simulink model "DTM_sim"  (R2024b)
settings: Solver=ode3  StartTime=0.0  StopTime=time_simulated  FixedStep=time_step_size  RelTol=1e-3
values from neighbouring files (symbols this model uses):
  a = 0.276626506024    [Fufy.mat]    (also in STMDrift.m = 1.347; Trajectory_LQR_double_track_Workspace_Phase_Plane_16_06.m = l-b; initParam.m = l-b)
  Ackerman_front = 0    [Fufy.mat]
  Ackerman_rear = 0    [Fufy.mat]
  b = 0.283373493976    [Fufy.mat]    (also in STMDrift.m = 1.393; Trajectory_LQR_double_track_Workspace_Phase_Plane_16_06.m = l/2; initParam.m = l/2)
  constant_force = 9    [runSIM.m]
  constant_steer = deg2rad(15)    [runSIM.m]
  d = 0    [Fufy.mat]
  d_front = 0    [Fufy.mat]
  d_rear = 0    [Fufy.mat]
  g = 9.81    [Fufy.mat]    (also in STMDrift.m)
  gamma = pi/2    (= 1.57079632679)    [Trajectory_LQR_double_track_Workspace_Phase_Plane_16_06.m]    (also in initParam.m; runSIM.m = 0)
  h = 0.128945128333    [Fufy.mat]    (also in STMDrift.m = [v;       beta;       d_delta;       d_Fx]; Trajectory_LQR_double_track_Workspace_Phase_Plane_16_06.m = (Fz_rear*l/(Fz_Tot)-(l-b))*cot(asin(H/l))+(R_r+R_f)/2; initParam.m = (Fz_Rear*l/(Fz_Tot)-(l-b))*cot(asin(H/l))+(R_r+R_f)/2)
  I_wheel = 0.002933125    [Fufy.mat]
  J_CoG = 1.30125108434    [Fufy.mat]    (also in Trajectory_LQR_double_track_Workspace_Phase_Plane_16_06.m = 9.4*a^2+9.4*b^2; initParam.m = 9.4*a^2+9.4*b^2)
  k_roll_front = 1    [Fufy.mat]
  k_roll_rear = 1    [Fufy.mat]
  l = 0.56    [Fufy.mat]
  m = 16.6    [Fufy.mat]    (also in STMDrift.m = 2137.3; Trajectory_LQR_double_track_Workspace_Phase_Plane_16_06.m = 18.8; initParam.m = 18.8)
  R_f = 0.095    [Fufy.mat]
  R_fl = R_f    [Trajectory_LQR_double_track_Workspace_Phase_Plane_16_06.m]    (also in initParam.m)
  R_fr = R_f    [Trajectory_LQR_double_track_Workspace_Phase_Plane_16_06.m]    (also in initParam.m)
  R_r = 0.095    [Fufy.mat]
  R_rl = R_r    [Trajectory_LQR_double_track_Workspace_Phase_Plane_16_06.m]    (also in initParam.m)
  R_rr = R_r    [Trajectory_LQR_double_track_Workspace_Phase_Plane_16_06.m]    (also in initParam.m)
  steering_ratio_f = 0.6    [Fufy.mat]
  steering_ratio_r = 0    [Fufy.mat]
  t_front = t    [Trajectory_LQR_double_track_Workspace_Phase_Plane_16_06.m]    (also in initParam.m)
  t_rear = t    [Trajectory_LQR_double_track_Workspace_Phase_Plane_16_06.m]    (also in initParam.m)
  Toe_fl = -0*pi/180    (= 0)    [Trajectory_LQR_double_track_Workspace_Phase_Plane_16_06.m]    (also in initParam.m)
  Toe_fr = -Toe_fl    (= 0)    [Trajectory_LQR_double_track_Workspace_Phase_Plane_16_06.m]    (also in initParam.m)
  Toe_rl = 0*pi/180    (= 0)    [Trajectory_LQR_double_track_Workspace_Phase_Plane_16_06.m]    (also in initParam.m)
  Toe_rr = -Toe_rl    (= 0)    [Trajectory_LQR_double_track_Workspace_Phase_Plane_16_06.m]    (also in initParam.m)
  u0 = 0    [Trajectory_LQR_double_track_Workspace_Phase_Plane_16_06.m]    (also in runSIM.m = 1)
  v0 = 0    [Trajectory_LQR_double_track_Workspace_Phase_Plane_16_06.m]    (also in runSIM.m = 8)
  yaw_rate0 = 0    [Trajectory_LQR_double_track_Workspace_Phase_Plane_16_06.m]    (also in runSIM.m = deg2rad(15))
undefined symbols (not defined in the file or in its folder): angular_speed_fl0, angular_speed_fr0, angular_speed_rl0, angular_speed_rr0, Fz_fl, Fz_fr, Fz_rl, Fz_rr
libraries: simulink_extras x1
settings Model: Creator=pc  LastModifiedBy=mg

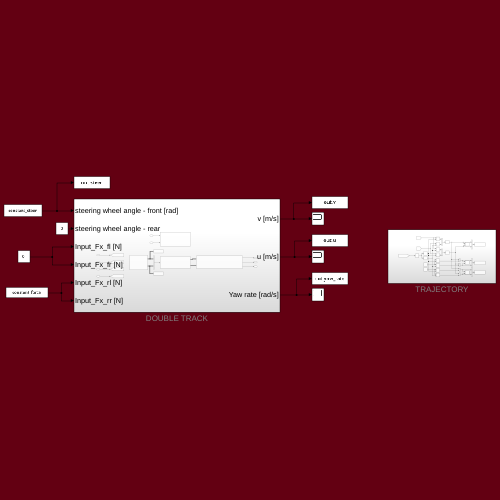
[thumbnail: Simulink's stored preview of the top-level diagram]
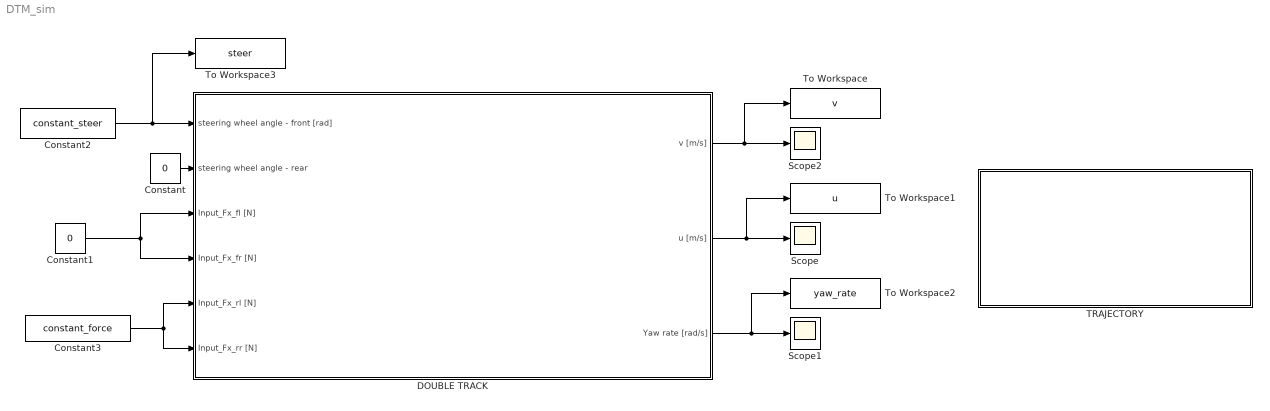
== system DTM_sim ==
  Constant : Constant  Value=0
  Constant1 : Constant  Value=0
  Constant2 : Constant  Value=constant_steer
  Constant3 : Constant  Value=constant_force
  DOUBLE TRACK : Subsystem
  Scope : Scope
  Scope1 : Scope
  Scope2 : Scope
  TRAJECTORY : Subsystem
  To Workspace : ToWorkspace  VariableName=v  SampleTime=-1
  To Workspace1 : ToWorkspace  VariableName=u  SampleTime=-1
  To Workspace2 : ToWorkspace  VariableName=yaw_rate  SampleTime=-1
  To Workspace3 : ToWorkspace  VariableName=steer  SampleTime=-1
  wires:
  Constant/1 -> DOUBLE TRACK/2(steering wheel angle - rear)
  Constant1/1 -> DOUBLE TRACK/4(Input_Fx_fr [N]), DOUBLE TRACK/3(Input_Fx_fl [N])
  DOUBLE TRACK/2(u [m/s]) -> To Workspace1/1, Scope/1
  DOUBLE TRACK/3(Yaw rate [rad/s]) -> To Workspace2/1, Scope1/1
  DOUBLE TRACK/1(v [m/s]) -> To Workspace/1, Scope2/1
  Constant2/1 -> To Workspace3/1, DOUBLE TRACK/1(steering wheel angle - front [rad])
  Constant3/1 -> DOUBLE TRACK/6(Input_Fx_rr [N]), DOUBLE TRACK/5(Input_Fx_rl [N])

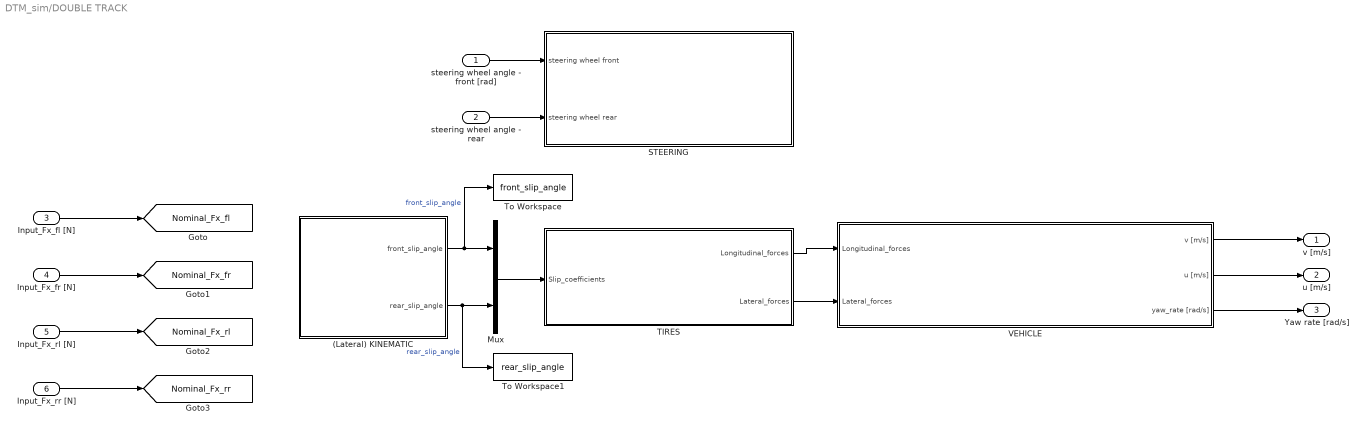
== system DTM_sim/DOUBLE TRACK ==
  steering wheel angle - front [rad] : Inport
  steering wheel angle - rear : Inport  Port=2
  Input_Fx_fl [N] : Inport  Port=3
  Input_Fx_fr [N] : Inport  Port=4
  Input_Fx_rl [N] : Inport  Port=5
  Input_Fx_rr [N] : Inport  Port=6
  (Lateral) KINEMATIC : Subsystem
  Mux : Mux  Inputs=2
  STEERING : Subsystem
  TIRES : Subsystem
  To Workspace : ToWorkspace  VariableName=front_slip_angle  SampleTime=-1
  To Workspace1 : ToWorkspace  VariableName=rear_slip_angle  SampleTime=-1
  VEHICLE : Subsystem
  v [m/s] : Outport
  u [m/s] : Outport  Port=2
  Yaw rate [rad/s] : Outport  Port=3
  tag scope: Nominal_Fx_fl=global, Nominal_Fx_fr=global, Nominal_Fx_rl=global, Nominal_Fx_rr=global
  wires:
  steering wheel angle - front [rad]/1 -> STEERING/1(steering wheel front)
  steering wheel angle - rear/1 -> STEERING/2(steering wheel rear)
  Input_Fx_fl [N]/1 -> [Nominal_Fx_fl]
  Input_Fx_fr [N]/1 -> [Nominal_Fx_fr]
  Input_Fx_rl [N]/1 -> [Nominal_Fx_rl]
  Input_Fx_rr [N]/1 -> [Nominal_Fx_rr]
  (Lateral) KINEMATIC/2(rear_slip_angle) -> To Workspace1/1, Mux/2  "rear_slip_angle"
  (Lateral) KINEMATIC/1(front_slip_angle) -> To Workspace/1, Mux/1  "front_slip_angle"
  Mux/1 -> TIRES/1(Slip_coefficients)
  TIRES/1(Longitudinal_forces) -> VEHICLE/1(Longitudinal_forces)
  TIRES/2(Lateral_forces) -> VEHICLE/2(Lateral_forces)
  VEHICLE/3(yaw_rate [rad/s]) -> Yaw rate [rad/s]/1
  VEHICLE/2(u [m/s]) -> u [m/s]/1
  VEHICLE/1(v [m/s]) -> v [m/s]/1

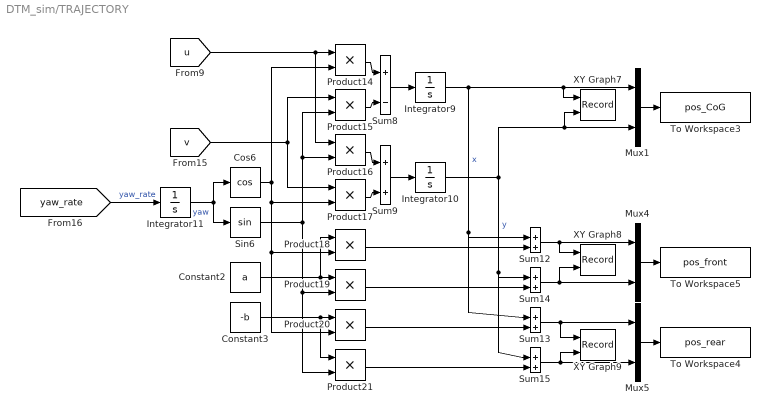
== system DTM_sim/TRAJECTORY ==
  Constant2 : Constant  Value=a
  Constant3 : Constant  Value=-b
  Cos6 : Trigonometry  Operator=cos
  Integrator10 : Integrator  InitialCondition=v0
  Integrator11 : Integrator  InitialCondition=gamma
  Integrator9 : Integrator  InitialCondition=u0
  Mux1 : Mux  Inputs=2
  Mux4 : Mux  Inputs=2
  Mux5 : Mux  Inputs=2
  Product{14..21} (8 alike) : Product
  Sin6 : Trigonometry
  Sum{9,12..15} (5 alike) : Sum  Inputs=+||+
  Sum8 : Sum  Inputs=+||-
  To Workspace3 : ToWorkspace  VariableName=pos_CoG  SampleTime=-1
  To Workspace4 : ToWorkspace  VariableName=pos_rear  SampleTime=-1
  To Workspace5 : ToWorkspace  VariableName=pos_front  SampleTime=-1
  XY Graph7 : Record  FileSettingsInternal="{\"entries\":[{\"content\":{\"excelSettings\":{\"content\":{},\"type\":\"Streamout.ExcelSettings\"}},\"type\":\"Streamout.FileSettingStorage\",\"uuid\":\"\"}],\"packageUris\":[\"http:\\/\\/schema.mathworks.com\\/mf0\\/streamout_blocks\\/R2020a\"],\"version\":\"1.0\"}"  Layout=[1 1]  SignalsInternal="{\"entries\":[{\"content\":{\"signals\":[{\"content\":{\"blockPath\":[],\"dimensions\":[1],\"domain\":\"\",\"lineColor\":\"#64d413\",\"lineWidth\":2,\"port\":1,\"signalID\":1,\"signalName\":\"MATLAB Function1\"},\"type\":\"RecordBlkView.Signal\",\"uuid\":\"\"},{\"content\":{\"blockPath\":[],\"dimensions\":[1],\"domain\":\"\",\"lineColor\":\"#ff13a6\",\"lineWidth\":2,\"port\":2,\"signalID\":2,\"signalName\":\"MATLAB Function\"},\"type\":\"RecordBlkView.Signal\",\"uuid\":\"\"}]},\"type\":\"RecordBlkView.InputSignals\",\"uuid\":\"\"}],\"packageUris\":[\"http:\\/\\/schema.mathworks.com\\/mf0\\/streamout_blocks\\/R2020a\"],\"version\":\"1.0\"}"  VisualizationBindings="{\"xyplotplugin\":{\"info\":[{\"series\":[],\"subplotID\":1}]}}"  CompatibilityTag=XY
  XY Graph8 : Record  FileSettingsInternal="{\"entries\":[{\"content\":{\"excelSettings\":{\"content\":{},\"type\":\"Streamout.ExcelSettings\"}},\"type\":\"Streamout.FileSettingStorage\",\"uuid\":\"\"}],\"packageUris\":[\"http:\\/\\/schema.mathworks.com\\/mf0\\/streamout_blocks\\/R2020a\"],\"version\":\"1.0\"}"  Layout=[1 1]  SignalsInternal="{\"entries\":[{\"content\":{\"signals\":[{\"content\":{\"blockPath\":[],\"dimensions\":[1],\"domain\":\"\",\"lineColor\":\"#64d413\",\"lineWidth\":2,\"port\":1,\"signalID\":1,\"signalName\":\"MATLAB Function1\"},\"type\":\"RecordBlkView.Signal\",\"uuid\":\"\"},{\"content\":{\"blockPath\":[],\"dimensions\":[1],\"domain\":\"\",\"lineColor\":\"#ff13a6\",\"lineWidth\":2,\"port\":2,\"signalID\":2,\"signalName\":\"MATLAB Function\"},\"type\":\"RecordBlkView.Signal\",\"uuid\":\"\"}]},\"type\":\"RecordBlkView.InputSignals\",\"uuid\":\"\"}],\"packageUris\":[\"http:\\/\\/schema.mathworks.com\\/mf0\\/streamout_blocks\\/R2020a\"],\"version\":\"1.0\"}"  VisualizationBindings="{\"xyplotplugin\":{\"info\":[{\"series\":[],\"subplotID\":1}]}}"  CompatibilityTag=XY
  XY Graph9 : Record  FileSettingsInternal="{\"entries\":[{\"content\":{\"excelSettings\":{\"content\":{},\"type\":\"Streamout.ExcelSettings\"}},\"type\":\"Streamout.FileSettingStorage\",\"uuid\":\"\"}],\"packageUris\":[\"http:\\/\\/schema.mathworks.com\\/mf0\\/streamout_blocks\\/R2020a\"],\"version\":\"1.0\"}"  Layout=[1 1]  SignalsInternal="{\"entries\":[{\"content\":{\"signals\":[{\"content\":{\"blockPath\":[],\"dimensions\":[1],\"domain\":\"\",\"lineColor\":\"#64d413\",\"lineWidth\":2,\"port\":1,\"signalID\":1,\"signalName\":\"MATLAB Function1\"},\"type\":\"RecordBlkView.Signal\",\"uuid\":\"\"},{\"content\":{\"blockPath\":[],\"dimensions\":[1],\"domain\":\"\",\"lineColor\":\"#ff13a6\",\"lineWidth\":2,\"port\":2,\"signalID\":2,\"signalName\":\"MATLAB Function\"},\"type\":\"RecordBlkView.Signal\",\"uuid\":\"\"}]},\"type\":\"RecordBlkView.InputSignals\",\"uuid\":\"\"}],\"packageUris\":[\"http:\\/\\/schema.mathworks.com\\/mf0\\/streamout_blocks\\/R2020a\"],\"version\":\"1.0\"}"  VisualizationBindings="{\"xyplotplugin\":{\"info\":[{\"series\":[],\"subplotID\":1}]}}"  CompatibilityTag=XY
  wires:
  Mux4/1 -> To Workspace5/1
  Mux5/1 -> To Workspace4/1
  Sum13/1 -> Mux5/1, XY Graph9/1
  Sum15/1 -> Mux5/2, XY Graph9/2
  Sum14/1 -> XY Graph8/2, Mux4/2
  Sum12/1 -> Mux4/1, XY Graph8/1
  Constant3/1 -> Product20/1, Product21/1
  Constant2/1 -> Product18/1, Product19/1
  Product20/1 -> Sum13/2
  Product21/1 -> Sum15/2
  Product19/1 -> Sum14/2
  Product18/1 -> Sum12/2
  Mux1/1 -> To Workspace3/1
  Sum9/1 -> Integrator10/1
  Sum8/1 -> Integrator9/1
  [v] -> Product17/1, Product15/1
  Product16/1 -> Sum9/1
  Product17/1 -> Sum9/2
  Product15/1 -> Sum8/2
  Sin6/1 -> Product19/2, Product21/2, Product15/2, Product16/2
  Product14/1 -> Sum8/1
  [u] -> Product14/1, Product16/1
  Cos6/1 -> Product14/2, Product17/2, Product18/2, Product20/2
  Integrator11/1 -> Cos6/1, Sin6/1  "yaw"
  Integrator10/1 -> Mux1/2, XY Graph7/2, Sum14/1, Sum15/1  "y"
  Integrator9/1 -> XY Graph7/1, Mux1/1, Sum12/1, Sum13/1  "x"
  [yaw_rate] -> Integrator11/1  "yaw_rate"

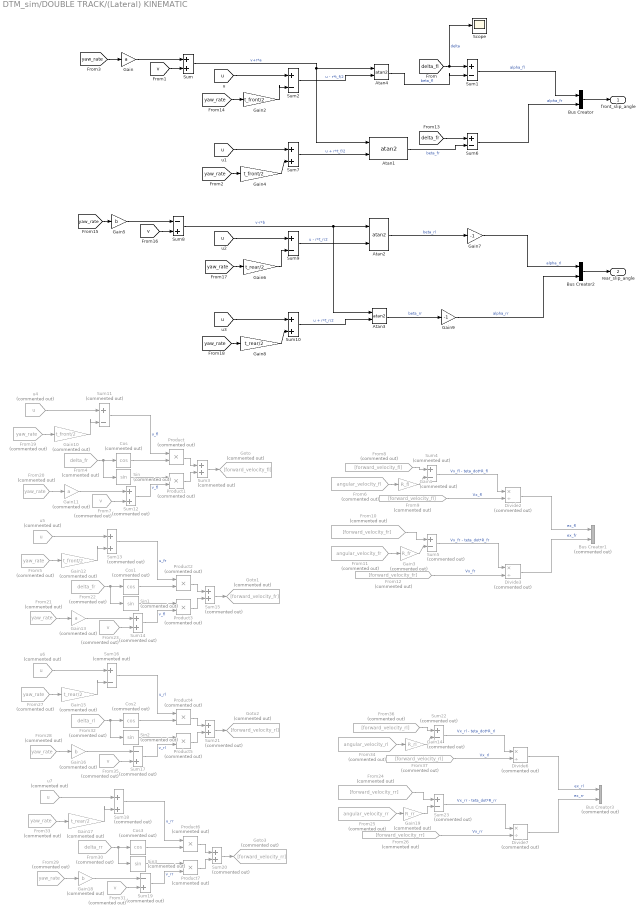
== system DTM_sim/DOUBLE TRACK/(Lateral) KINEMATIC ==
  Atan{1..4} (4 alike) : Trigonometry  Operator=atan2
  Bus Creator : BusCreator  Inputs=2
  Bus Creator1 : BusCreator  Commented=on  Inputs=2
  Bus Creator2 : BusCreator  Inputs=2
  Bus Creator3 : BusCreator  Commented=on  Inputs=2
  Cos{,1..3} (4 alike) : Trigonometry  Commented=on  Operator=cos
  Divide{2..3,6..7} (4 alike) : Product  Commented=on  Inputs=*/
  From10 : From  Commented=on  GotoTag=forward_velocity_fr
  From11 : From  Commented=on  GotoTag=angular_velocity_fr  TagVisibility=global
  From12 : From  Commented=on  GotoTag=forward_velocity_fr
  From{5,19..21,27..29,33} (8 alike) : From  Commented=on  GotoTag=yaw_rate  TagVisibility=global
  From22 : From  Commented=on  GotoTag=delta_fr  TagVisibility=global
  From{7,23,31,35} (4 alike) : From  Commented=on  GotoTag=v  TagVisibility=global
  From24 : From  Commented=on  GotoTag=forward_velocity_rr
  From25 : From  Commented=on  GotoTag=angular_velocity_rr  TagVisibility=global
  From26 : From  Commented=on  GotoTag=forward_velocity_rr
  From30 : From  Commented=on  GotoTag=delta_rr  TagVisibility=global
  From32 : From  Commented=on  GotoTag=delta_rl  TagVisibility=global
  From34 : From  Commented=on  GotoTag=angular_velocity_rl  TagVisibility=global
  From36 : From  Commented=on  GotoTag=forward_velocity_rl
  From37 : From  Commented=on  GotoTag=forward_velocity_rl
  From4 : From  Commented=on  GotoTag=delta_fr  TagVisibility=global
  From6 : From  Commented=on  GotoTag=angular_velocity_fl  TagVisibility=global
  From8 : From  Commented=on  GotoTag=forward_velocity_fl
  From9 : From  Commented=on  GotoTag=forward_velocity_fl
  Gain : Gain  Gain=a
  Gain1 : Gain  Commented=on  Gain=R_fl
  Gain10 : Gain  Commented=on  Gain=t_front/2
  Gain11 : Gain  Commented=on  Gain=a
  Gain12 : Gain  Commented=on  Gain=t_front/2
  Gain13 : Gain  Commented=on  Gain=a
  Gain14 : Gain  Commented=on  Gain=R_rl
  Gain15 : Gain  Commented=on  Gain=t_rear/2
  Gain16 : Gain  Commented=on  Gain=b
  Gain17 : Gain  Commented=on  Gain=t_rear/2
  Gain18 : Gain  Commented=on  Gain=b
  Gain19 : Gain  Commented=on  Gain=R_rr
  Gain2 : Gain  Gain=t_front/2
  Gain3 : Gain  Commented=on  Gain=R_fr
  Gain4 : Gain  Gain=t_front/2
  Gain5 : Gain  Gain=b
  Gain6 : Gain  Gain=t_rear/2
  Gain7 : Gain  Gain=-1
  Gain8 : Gain  Gain=t_rear/2
  Gain9 : Gain  Gain=-1
  Goto : Goto  Commented=on  GotoTag=forward_velocity_fl
  Goto1 : Goto  Commented=on  GotoTag=forward_velocity_fr
  Goto2 : Goto  Commented=on  GotoTag=forward_velocity_rl
  Goto3 : Goto  Commented=on  GotoTag=forward_velocity_rr
  Product{,1..7} (8 alike) : Product  Commented=on
  Scope : Scope
  Sin{,1..3} (4 alike) : Trigonometry  Commented=on
  Sum : Sum  Inputs=||+|||+||
  Sum1 : Sum  Inputs=||+||-||
  Sum10 : Sum  Inputs=||+|||+||
  Sum11 : Sum  Commented=on  Inputs=||+|||-||
  Sum{12..14,18} (4 alike) : Sum  Commented=on  Inputs=||+|||+||
  Sum{3,15,20..21} (4 alike) : Sum  Commented=on  Inputs=||+||+||
  Sum16 : Sum  Commented=on  Inputs=||+|||-||
  Sum17 : Sum  Commented=on  Inputs=||-|||+||
  Sum19 : Sum  Commented=on  Inputs=||-|||+||
  Sum2 : Sum  Inputs=||+|||-||
  Sum{4..5,22..23} (4 alike) : Sum  Commented=on  Inputs=||+||-||
  Sum6 : Sum  Inputs=||+||-||
  Sum7 : Sum  Inputs=||+|||+||
  Sum8 : Sum  Inputs=||-|||+||
  Sum9 : Sum  Inputs=||+|||-||
  u{4..7} (4 alike) : From  Commented=on  GotoTag=u  TagVisibility=global
  front_slip_angle : Outport
  rear_slip_angle : Outport  Port=2
  wires:
  Sum/1 -> Atan4/1, Atan1/1  "v+r*a"
  Atan4/1 -> Sum1/2  "beta_fl"
  [delta_fl] -> Scope/1, Sum1/1  "delta"
  [yaw_rate] -> Gain/1
  Atan1/1 -> Sum6/2  "beta_fr"
  Bus Creator/1 -> front_slip_angle/1
  Sum7/1 -> Atan1/2  "u + r*t_f/2"
  [v] -> Sum/2
  Gain/1 -> Sum/1
  From4/1 -> Sin/1, Cos/1
  Cos/1 -> Product/2
  Sin/1 -> Product1/1
  From6/1 -> Gain1/1
  Gain1/1 -> Sum4/2
  Sum4/1 -> Divide2/1  "Vx_fl - teta_dot*R_fl"
  Product1/1 -> Sum3/2
  Product/1 -> Sum3/1
  Sum3/1 -> Goto/1
  From8/1 -> Sum4/1
  From9/1 -> Divide2/2  "Vx_fl"
  Divide2/1 -> Bus Creator1/1  "ex_fl"
  Gain3/1 -> Sum5/2
  From11/1 -> Gain3/1
  From10/1 -> Sum5/1
  Sum5/1 -> Divide3/1  "Vx_fr - teta_dot*R_fr"
  From12/1 -> Divide3/2  "Vx_fr"
  Divide3/1 -> Bus Creator1/2  "ex_fr"
  Sum6/1 -> Bus Creator/2  "alpha_fr"
  [delta_fr] -> Sum6/1
  [u] -> Sum2/1
  Sum2/1 -> Atan4/2  "u - r*t_f/2"
  [yaw_rate] -> Gain2/1
  Gain2/1 -> Sum2/2
  [u] -> Sum7/1
  [yaw_rate] -> Gain4/1
  Gain4/1 -> Sum7/2
  [yaw_rate] -> Gain5/1
  Gain5/1 -> Sum8/1
  [v] -> Sum8/2
  Gain6/1 -> Sum9/2
  [u] -> Sum9/1
  [yaw_rate] -> Gain6/1
  Sum9/1 -> Atan2/2  "u - r*t_r/2"
  Atan2/1 -> Gain7/1  "beta_rl"
  Gain7/1 -> Bus Creator2/1  "alpha_rl"
  [u] -> Sum10/1
  Sum10/1 -> Atan3/2  "u + r*t_r/2"
  Sum8/1 -> Atan3/1, Atan2/1  "v-r*b"
  [yaw_rate] -> Gain8/1
  Gain8/1 -> Sum10/2
  Atan3/1 -> Gain9/1  "beta_rr"
  Gain9/1 -> Bus Creator2/2  "alpha_rr"
  Bus Creator2/1 -> rear_slip_angle/1
  u4/1 -> Sum11/1
  From19/1 -> Gain10/1
  Sum11/1 -> Product/1  "u_fl"
  Gain10/1 -> Sum11/2
  Gain11/1 -> Sum12/1
  From20/1 -> Gain11/1
  From7/1 -> Sum12/2
  Sum12/1 -> Product1/2  "v_fl"
  Sum14/1 -> Product3/2  "v_fl"
  Sum13/1 -> Product2/1  "u_fr"
  Gain12/1 -> Sum13/2
  u5/1 -> Sum13/1
  From23/1 -> Sum14/2
  Gain13/1 -> Sum14/1
  From21/1 -> Gain13/1
  Product3/1 -> Sum15/2
  Product2/1 -> Sum15/1
  From5/1 -> Gain12/1
  Sin1/1 -> Product3/1
  Sum15/1 -> Goto1/1
  Cos1/1 -> Product2/2
  From22/1 -> Sin1/1, Cos1/1
  Sum17/1 -> Product5/2  "v_rl"
  Sum16/1 -> Product4/1  "u_rl"
  Product7/1 -> Sum20/2
  From30/1 -> Sin3/1, Cos3/1
  From33/1 -> Gain17/1
  Sin3/1 -> Product7/1
  Cos3/1 -> Product6/2
  From29/1 -> Gain18/1
  Sum18/1 -> Product6/1  "u_rr"
  Sum20/1 -> Goto3/1
  u7/1 -> Sum18/1
  Gain17/1 -> Sum18/2
  Gain15/1 -> Sum16/2
  u6/1 -> Sum16/1
  From35/1 -> Sum17/2
  Gain18/1 -> Sum19/1
  Gain16/1 -> Sum17/1
  From28/1 -> Gain16/1
  From34/1 -> Gain14/1
  Sum22/1 -> Divide6/1  "Vx_rl - teta_dot*R_rl"
  Divide6/1 -> Bus Creator3/1  "ex_rl"
  From31/1 -> Sum19/2
  Cos2/1 -> Product4/2
  Sum23/1 -> Divide7/1  "Vx_rr - teta_dot*R_rr"
  From26/1 -> Divide7/2  "Vx_rr"
  Gain19/1 -> Sum23/2
  From37/1 -> Divide6/2  "Vx_rl"
  Divide7/1 -> Bus Creator3/2  "ex_rr"
  From24/1 -> Sum23/1
  Product5/1 -> Sum21/2
  From25/1 -> Gain19/1
  Product4/1 -> Sum21/1
  From27/1 -> Gain15/1
  Sin2/1 -> Product5/1
  Sum21/1 -> Goto2/1
  From36/1 -> Sum22/1
  Product6/1 -> Sum20/1
  From32/1 -> Sin2/1, Cos2/1
  Sum19/1 -> Product7/2  "v_rr"
  Gain14/1 -> Sum22/2
  Sum1/1 -> Bus Creator/1  "alpha_fl"

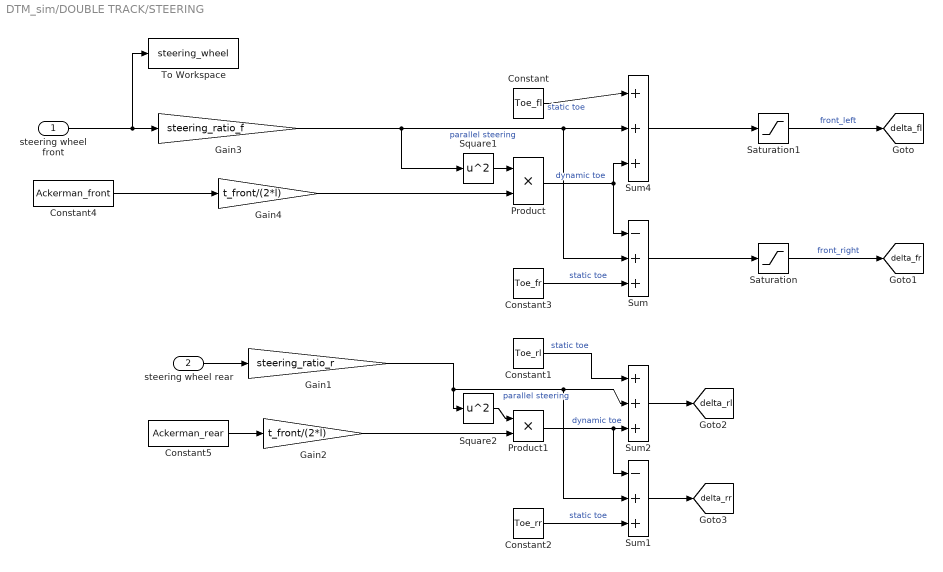
== system DTM_sim/DOUBLE TRACK/STEERING ==
  steering wheel front : Inport
  steering wheel rear : Inport  Port=2
  Constant : Constant  Value=Toe_fl
  Constant1 : Constant  Value=Toe_rl
  Constant2 : Constant  Value=Toe_rr
  Constant3 : Constant  Value=Toe_fr
  Constant4 : Constant  Value=Ackerman_front
  Constant5 : Constant  Value=Ackerman_rear
  Gain1 : Gain  Gain=steering_ratio_r
  Gain2 : Gain  Gain=t_front/(2*l)
  Gain3 : Gain  Gain=steering_ratio_f
  Gain4 : Gain  Gain=t_front/(2*l)
  Product : Product
  Product1 : Product
  Saturation : Saturate  UpperLimit=deg2rad(0.6*(84-47))  LowerLimit=deg2rad(0.6*(47-84))
  Saturation1 : Saturate  UpperLimit=deg2rad(0.6*(84-47))  LowerLimit=deg2rad(0.6*(47-84))
  Square1 : Math  Operator=square
  Square2 : Math  Operator=square
  Sum : Sum  Inputs=|-||||+||||+|
  Sum1 : Sum  Inputs=|-||||+||||+|
  Sum2 : Sum  Inputs=|+||||+||||+|
  Sum4 : Sum  Inputs=|+||||+||||+|
  To Workspace : ToWorkspace  VariableName=steering_wheel  SaveFormat=Structure With Time  SampleTime=-1
  tag scope: delta_fl=global, delta_fr=global, delta_rl=global, delta_rr=global
  wires:
  Constant4/1 -> Gain4/1
  Constant3/1 -> Sum/3  "static toe"
  Constant/1 -> Sum4/1  "static toe"
  steering wheel front/1 -> To Workspace/1, Gain3/1
  Product/1 -> Sum/1, Sum4/3  "dynamic toe"
  Gain3/1 -> Sum/2, Sum4/2, Square1/1  "parallel steering"
  Gain4/1 -> Product/2
  Square1/1 -> Product/1
  Constant1/1 -> Sum2/1  "static toe"
  Gain1/1 -> Square2/1, Sum1/2, Sum2/2  "parallel steering"
  steering wheel rear/1 -> Gain1/1
  Square2/1 -> Product1/1
  Sum1/1 -> [delta_rr]
  Product1/1 -> Sum1/1, Sum2/3  "dynamic toe"
  Gain2/1 -> Product1/2
  Sum2/1 -> [delta_rl]
  Constant5/1 -> Gain2/1
  Constant2/1 -> Sum1/3  "static toe"
  Sum4/1 -> Saturation1/1
  Saturation/1 -> [delta_fr]  "front_right"
  Saturation1/1 -> [delta_fl]  "front_left"
  Sum/1 -> Saturation/1

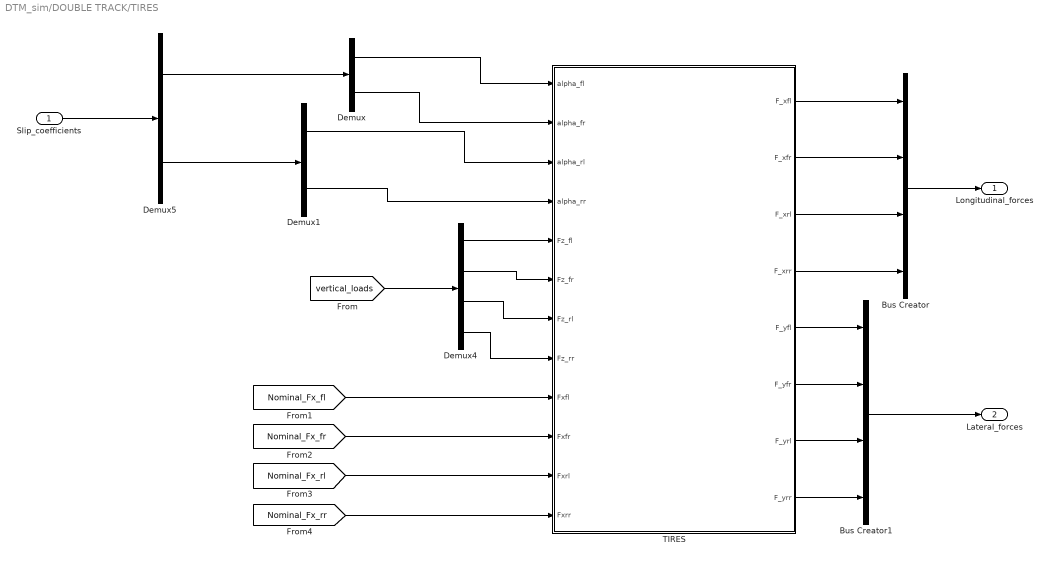
== system DTM_sim/DOUBLE TRACK/TIRES ==
  Slip_coefficients : Inport
  Bus Creator : BusCreator  Inputs=4
  Bus Creator1 : BusCreator  Inputs=4
  Demux : Demux  Outputs=2
  Demux1 : Demux  Outputs=2
  Demux4 : Demux
  Demux5 : Demux  Outputs=2
  TIRES : MATLAB Function  TreatAsAtomicUnit=on
  Longitudinal_forces : Outport
  Lateral_forces : Outport  Port=2
  wires:
  Bus Creator1/1 -> Lateral_forces/1
  Bus Creator/1 -> Longitudinal_forces/1
  Slip_coefficients/1 -> Demux5/1
  [vertical_loads] -> Demux4/1
  TIRES/1(F_xfl) -> Bus Creator/1
  TIRES/2(F_xfr) -> Bus Creator/2
  TIRES/3(F_xrl) -> Bus Creator/3
  TIRES/4(F_xrr) -> Bus Creator/4
  TIRES/5(F_yfl) -> Bus Creator1/1
  TIRES/6(F_yfr) -> Bus Creator1/2
  TIRES/7(F_yrl) -> Bus Creator1/3
  TIRES/8(F_yrr) -> Bus Creator1/4
  Demux/1 -> TIRES/1(alpha_fl)
  Demux/2 -> TIRES/2(alpha_fr)
  Demux1/1 -> TIRES/3(alpha_rl)
  Demux1/2 -> TIRES/4(alpha_rr)
  Demux4/1 -> TIRES/5(Fz_fl)
  Demux4/2 -> TIRES/6(Fz_fr)
  Demux4/3 -> TIRES/7(Fz_rl)
  Demux4/4 -> TIRES/8(Fz_rr)
  Demux5/2 -> Demux1/1
  Demux5/1 -> Demux/1
  [Nominal_Fx_fl] -> TIRES/9(Fxfl)
  [Nominal_Fx_fr] -> TIRES/10(Fxfr)
  [Nominal_Fx_rl] -> TIRES/11(Fxrl)
  [Nominal_Fx_rr] -> TIRES/12(Fxrr)

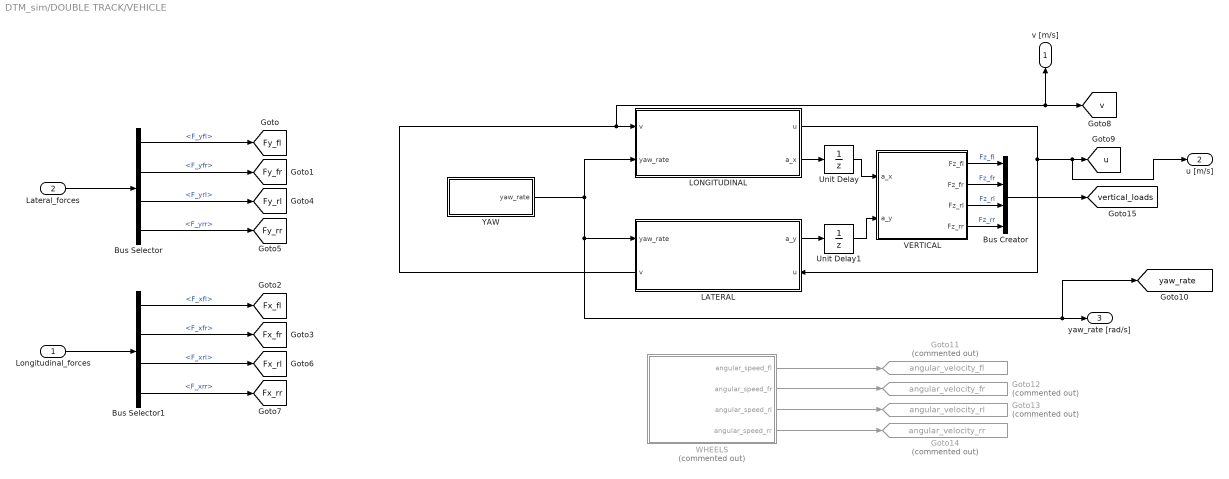
== system DTM_sim/DOUBLE TRACK/VEHICLE ==
  Longitudinal_forces : Inport
  Lateral_forces : Inport  Port=2
  Bus Creator : BusCreator  Inputs=Fz_fl,Fz_fr,Fz_rl,Fz_rr
  Bus Selector : BusSelector  OutputSignals=F_yfl,F_yfr,F_yrl,F_yrr
  Bus Selector1 : BusSelector  OutputSignals=F_xfl,F_xfr,F_xrl,F_xrr
  Goto11 : Goto  Commented=on  GotoTag=angular_velocity_fl  TagVisibility=global
  Goto12 : Goto  Commented=on  GotoTag=angular_velocity_fr  TagVisibility=global
  Goto13 : Goto  Commented=on  GotoTag=angular_velocity_rl  TagVisibility=global
  Goto14 : Goto  Commented=on  GotoTag=angular_velocity_rr  TagVisibility=global
  LATERAL : Subsystem
      settings: PortSchema="{\"entries\":[{\"content\":{\"sides\":[{\"content\":{\"connectorIds\":[\"In1\",\"Out2\"]},\"type\":\"ConnectorPlacement.EquallySpacedRectSide\",\"uuid\":\"6abf6559-6621-467b-b855-11099c66163f\"},{\"content\":{\"connectorIds\":[\"Out1\",\"In2\"],\"side\":\"RIGHT\"},\"type\":\"ConnectorPlacement.EquallySpacedRectSide\",\"uuid\":\"e2281ccf-38f1-4c2e-94ea-91f999c21e12\"},{\"content\":{\"side\":\"TOP\"},\"type\":\"ConnectorPlacement.EquallySpacedRectSide\",\"uuid\":\"84832623-c0ad-4def-a112-064fe8d35bcd\"}]},\"type\":\"ConnectorPlacement.EquallySpacedConnector\",\"uuid\":\"accfadac-0c65-44f3-8a84-674bad9770b1\"}],\"packageUris\":[\"http://schema.mathworks.com/mf0/Connector/R2020b\"],\"version\":\"1.0\"}"
  LONGITUDINAL : Subsystem
  Unit Delay : UnitDelay  SampleTime=-1  HasFrameUpgradeWarning=on
  Unit Delay1 : UnitDelay  SampleTime=-1  HasFrameUpgradeWarning=on
  VERTICAL : Subsystem
  WHEELS : Subsystem  Commented=on
  YAW : Subsystem
  v [m/s] : Outport
  u [m/s] : Outport  Port=2
  yaw_rate [rad/s] : Outport  Port=3
  tag scope: Fx_fl=global, Fx_fr=global, Fx_rl=global, Fx_rr=global, Fy_fl=global, Fy_fr=global, Fy_rl=global, Fy_rr=global, u=global, v=global, vertical_loads=global, yaw_rate=global
  wires:
  Lateral_forces/1 -> Bus Selector/1
  Bus Selector/1 -> [Fy_fl]  "<F_yfl>"
  Bus Selector/2 -> [Fy_fr]  "<F_yfr>"
  Longitudinal_forces/1 -> Bus Selector1/1
  Bus Selector1/2 -> [Fx_fr]  "<F_xfr>"
  Bus Selector/3 -> [Fy_rl]  "<F_yrl>"
  Bus Selector/4 -> [Fy_rr]  "<F_yrr>"
  Bus Selector1/3 -> [Fx_rl]  "<F_xrl>"
  Bus Selector1/4 -> [Fx_rr]  "<F_xrr>"
  LATERAL/2(v) -> v [m/s]/1, [v], LONGITUDINAL/1(v)
  YAW/1(yaw_rate) -> LONGITUDINAL/2(yaw_rate), [yaw_rate], yaw_rate [rad/s]/1, LATERAL/1(yaw_rate)
  LONGITUDINAL/1(u) -> u [m/s]/1, [u], LATERAL/2(u)
  LONGITUDINAL/2(a_x) -> Unit Delay/1
  LATERAL/1(a_y) -> Unit Delay1/1
  VERTICAL/1(Fz_fl) -> Bus Creator/1  "Fz_fl"
  VERTICAL/2(Fz_fr) -> Bus Creator/2  "Fz_fr"
  VERTICAL/3(Fz_rl) -> Bus Creator/3  "Fz_rl"
  VERTICAL/4(Fz_rr) -> Bus Creator/4  "Fz_rr"
  Bus Creator/1 -> [vertical_loads]
  WHEELS/1(angular_speed_fl) -> Goto11/1
  WHEELS/2(angular_speed_fr) -> Goto12/1
  WHEELS/3(angular_speed_rl) -> Goto13/1
  WHEELS/4(angular_speed_rr) -> Goto14/1
  Unit Delay/1 -> VERTICAL/1(a_x)
  Unit Delay1/1 -> VERTICAL/2(a_y)
  Bus Selector1/1 -> [Fx_fl]  "<F_xfl>"

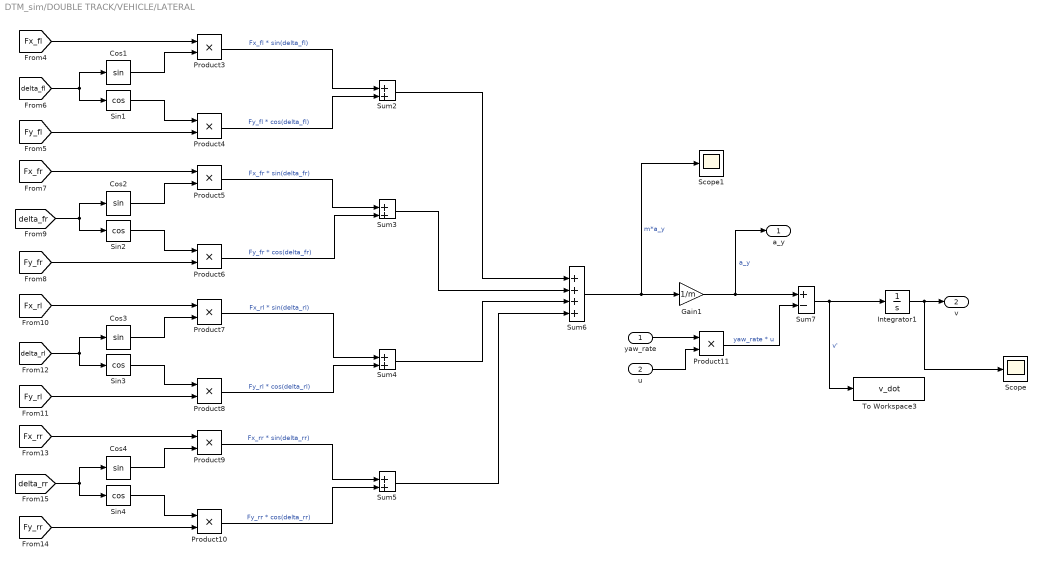
== system DTM_sim/DOUBLE TRACK/VEHICLE/LATERAL ==
  yaw_rate : Inport
  u : Inport  Port=2
  Cos{1..4} (4 alike) : Trigonometry
  Gain1 : Gain  Gain=1/m
  Integrator1 : Integrator  InitialCondition=v0
  Product{3..11} (9 alike) : Product
  Scope : Scope
  Scope1 : Scope
  Sin{1..4} (4 alike) : Trigonometry  Operator=cos
  Sum{2..5} (4 alike) : Sum  Inputs=|+||+|
  Sum6 : Sum  Inputs=|+|||+|||+|||+|
  Sum7 : Sum  Inputs=||+||-||
  To Workspace3 : ToWorkspace  VariableName=v_dot  SampleTime=-1
  a_y : Outport
  v : Outport  Port=2
  wires:
  [Fy_fl] -> Product4/2
  [Fx_fl] -> Product3/1
  Product4/1 -> Sum2/2  "Fy_fl * cos(delta_fl)"
  [delta_fl] -> Sin1/1, Cos1/1
  Cos1/1 -> Product3/2
  Product3/1 -> Sum2/1  "Fx_fl * sin(delta_fl)"
  Sin1/1 -> Product4/1
  [Fx_fr] -> Product5/1
  Cos2/1 -> Product5/2
  Sin2/1 -> Product6/1
  [delta_fr] -> Sin2/1, Cos2/1
  Product5/1 -> Sum3/1  "Fx_fr * sin(delta_fr)"
  [Fy_fr] -> Product6/2
  Product6/1 -> Sum3/2  "Fy_fr * cos(delta_fr)"
  [Fx_rl] -> Product7/1
  Sin3/1 -> Product8/1
  [delta_rl] -> Sin3/1, Cos3/1
  Product10/1 -> Sum5/2  "Fy_rr * cos(delta_rr)"
  [Fy_rr] -> Product10/2
  Product9/1 -> Sum5/1  "Fx_rr * sin(delta_rr)"
  Cos3/1 -> Product7/2
  Cos4/1 -> Product9/2
  Sin4/1 -> Product10/1
  [Fx_rr] -> Product9/1
  Product7/1 -> Sum4/1  "Fx_rl * sin(delta_rl)"
  [Fy_rl] -> Product8/2
  Product8/1 -> Sum4/2  "Fy_rl * cos(delta_rl)"
  [delta_rr] -> Sin4/1, Cos4/1
  Sum2/1 -> Sum6/1
  Sum3/1 -> Sum6/2
  Sum4/1 -> Sum6/3
  Sum5/1 -> Sum6/4
  Sum6/1 -> Scope1/1, Gain1/1  "m*a_y"
  yaw_rate/1 -> Product11/1
  u/1 -> Product11/2
  Product11/1 -> Sum7/2  "yaw_rate * u"
  Sum7/1 -> To Workspace3/1, Integrator1/1  "v'"
  Integrator1/1 -> Scope/1, v/1
  Gain1/1 -> a_y/1, Sum7/1  "a_y"

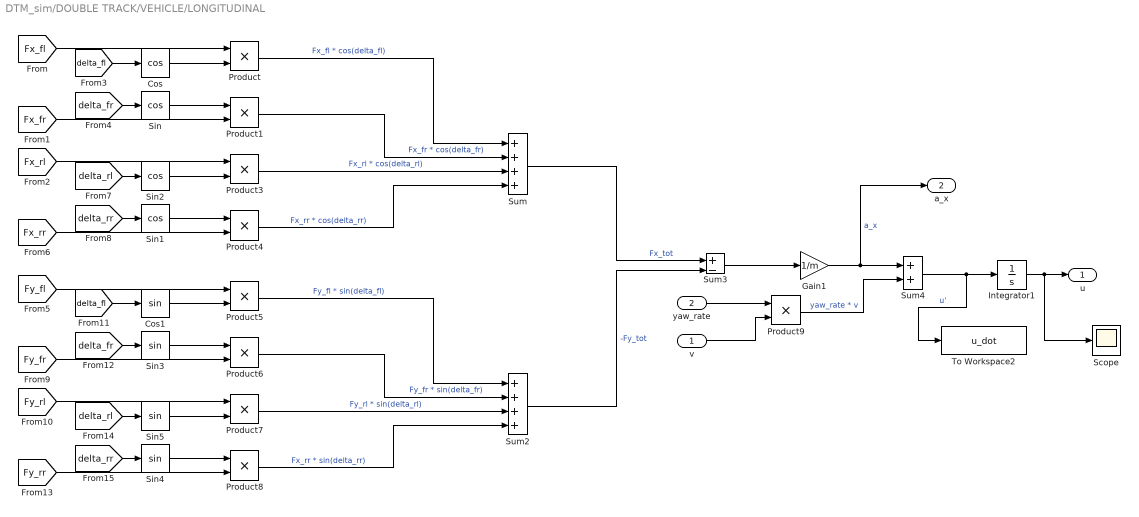
== system DTM_sim/DOUBLE TRACK/VEHICLE/LONGITUDINAL ==
  v : Inport
  yaw_rate : Inport  Port=2
  Cos : Trigonometry  Operator=cos
  Cos1 : Trigonometry
  Gain1 : Gain  Gain=1/m
  Integrator1 : Integrator  InitialCondition=u0
  Product{,1,3..9} (9 alike) : Product
  Scope : Scope
  Sin : Trigonometry  Operator=cos
  Sin1 : Trigonometry  Operator=cos
  Sin2 : Trigonometry  Operator=cos
  Sin3 : Trigonometry
  Sin4 : Trigonometry
  Sin5 : Trigonometry
  Sum : Sum  Inputs=||+||+||+||+||
  Sum2 : Sum  Inputs=||+||+||+||+||
  Sum3 : Sum  Inputs=+||-
  Sum4 : Sum  Inputs=||+||+||
  To Workspace2 : ToWorkspace  VariableName=u_dot  SampleTime=-1
  u : Outport
  a_x : Outport  Port=2
  wires:
  [Fx_fl] -> Product/1
  Cos/1 -> Product/2
  [Fx_fr] -> Product1/2
  Sin/1 -> Product1/1
  Product/1 -> Sum/1  "Fx_fl * cos(delta_fl)"
  Product1/1 -> Sum/2  "Fx_fr * cos(delta_fr)"
  [delta_fl] -> Cos/1
  [delta_fr] -> Sin/1
  [delta_rl] -> Sin2/1
  Sin2/1 -> Product3/2
  [Fx_rl] -> Product3/1
  [Fx_rr] -> Product4/2
  Sin1/1 -> Product4/1
  [delta_rr] -> Sin1/1
  Product3/1 -> Sum/3  "Fx_rl * cos(delta_rl)"
  Product4/1 -> Sum/4  "Fx_rr * cos(delta_rr)"
  Sum/1 -> Sum3/1  "Fx_tot"
  Sum2/1 -> Sum3/2  "-Fy_tot"
  Product8/1 -> Sum2/4  "Fx_rr * sin(delta_rr)"
  [delta_rl] -> Sin5/1
  [delta_rr] -> Sin4/1
  [Fy_rr] -> Product8/2
  [delta_fl] -> Cos1/1
  [Fy_fl] -> Product5/1
  Sin4/1 -> Product8/1
  Sin3/1 -> Product6/1
  Product5/1 -> Sum2/1  "Fy_fl * sin(delta_fl)"
  [Fy_fr] -> Product6/2
  [delta_fr] -> Sin3/1
  [Fy_rl] -> Product7/1
  Cos1/1 -> Product5/2
  Sin5/1 -> Product7/2
  Product7/1 -> Sum2/3  "Fy_rl * sin(delta_rl)"
  Product6/1 -> Sum2/2  "Fy_fr * sin(delta_fr)"
  Sum3/1 -> Gain1/1
  Gain1/1 -> a_x/1, Sum4/1  "a_x"
  Product9/1 -> Sum4/2  "yaw_rate * v"
  v/1 -> Product9/2
  yaw_rate/1 -> Product9/1
  Integrator1/1 -> Scope/1, u/1
  Sum4/1 -> To Workspace2/1, Integrator1/1  "u'"

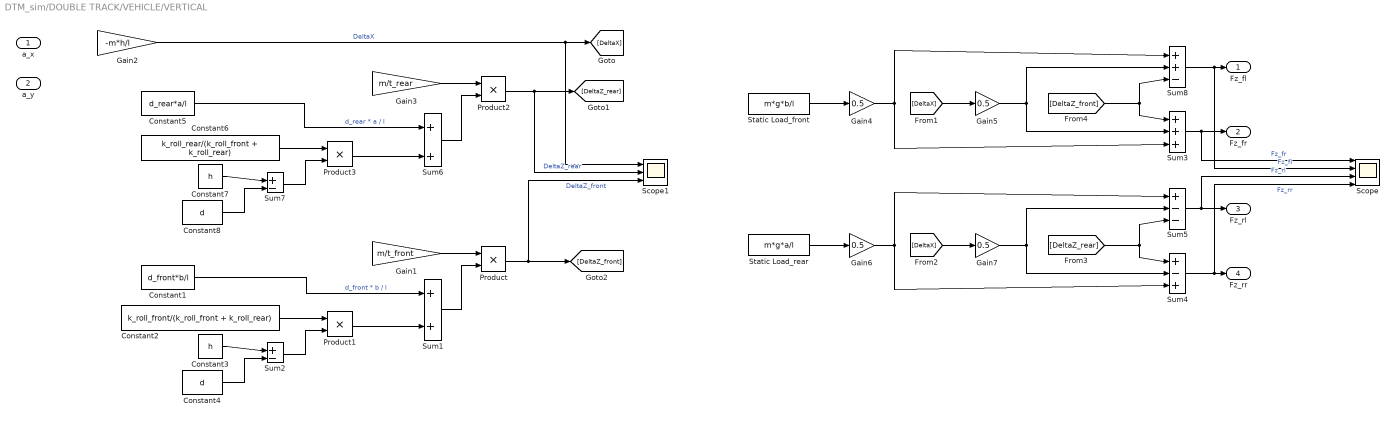
== system DTM_sim/DOUBLE TRACK/VEHICLE/VERTICAL ==
  a_x : Inport
  a_y : Inport  Port=2
  Constant1 : Constant  Value=d_front*b/l
  Constant2 : Constant  Value=k_roll_front/(k_roll_front + k_roll_rear)
  Constant3 : Constant  Value=h
  Constant4 : Constant  Value=d
  Constant5 : Constant  Value=d_rear*a/l
  Constant6 : Constant  Value=k_roll_rear/(k_roll_front + k_roll_rear)
  Constant7 : Constant  Value=h
  Constant8 : Constant  Value=d
  Gain1 : Gain  Gain=m/t_front
  Gain2 : Gain  Gain=-m*h/l
  Gain3 : Gain  Gain=m/t_rear
  Gain{4..7} (4 alike) : Gain  Gain=0.5
  Product{,1..3} (4 alike) : Product
  Scope : Scope  NumInputPorts=4
  Scope1 : Scope  NumInputPorts=3
  Static Load_front : Constant  Value=m*g*b/l
  Static Load_rear : Constant  Value=m*g*a/l
  Sum1 : Sum  Inputs=|+|||+|
  Sum2 : Sum  Inputs=|+||-|
  Sum3 : Sum  Inputs=|+|||+|||+|
  Sum4 : Sum  Inputs=|+|||-|||+|
  Sum5 : Sum  Inputs=|+|||-|||-|
  Sum6 : Sum  Inputs=|+|||+|
  Sum7 : Sum  Inputs=|+||-|
  Sum8 : Sum  Inputs=|+|||+|||-|
  Fz_fl : Outport
  Fz_fr : Outport  Port=2
  Fz_rl : Outport  Port=3
  Fz_rr : Outport  Port=4
  wires:
  Gain1/1 -> Product/1
  Sum1/1 -> Product/2
  Constant1/1 -> Sum1/1  "d_front * b / l"
  Constant2/1 -> Product1/1
  Product1/1 -> Sum1/2
  Sum2/1 -> Product1/2
  Constant3/1 -> Sum2/1
  Constant4/1 -> Sum2/2
  Product/1 -> Scope1/3, [DeltaZ_front]  "DeltaZ_front"
  Product2/1 -> Scope1/2, [DeltaZ_rear]  "DeltaZ_rear"
  Constant8/1 -> Sum7/2
  Gain3/1 -> Product2/1
  Product3/1 -> Sum6/2
  Sum7/1 -> Product3/2
  Constant6/1 -> Product3/1
  Constant5/1 -> Sum6/1  "d_rear * a / l"
  Sum6/1 -> Product2/2
  Constant7/1 -> Sum7/1
  Gain2/1 -> Scope1/1, [DeltaX]  "DeltaX"
  Sum5/1 -> Scope/3, Fz_rl/1  "Fz_rl"
  Static Load_rear/1 -> Gain6/1
  Sum4/1 -> Scope/4, Fz_rr/1  "Fz_rr"
  [DeltaX] -> Gain7/1
  [DeltaZ_rear] -> Sum5/3, Sum4/1
  Gain6/1 -> Sum5/1, Sum4/3
  Gain7/1 -> Sum5/2, Sum4/2
  Sum8/1 -> Scope/2, Fz_fl/1  "Fz_fl"
  [DeltaX] -> Gain5/1
  Sum3/1 -> Scope/1, Fz_fr/1  "Fz_fr"
  Gain4/1 -> Sum8/1, Sum3/3
  [DeltaZ_front] -> Sum8/3, Sum3/1
  Gain5/1 -> Sum8/2, Sum3/2
  Static Load_front/1 -> Gain4/1
  ? -> Gain1/1, Gain3/1

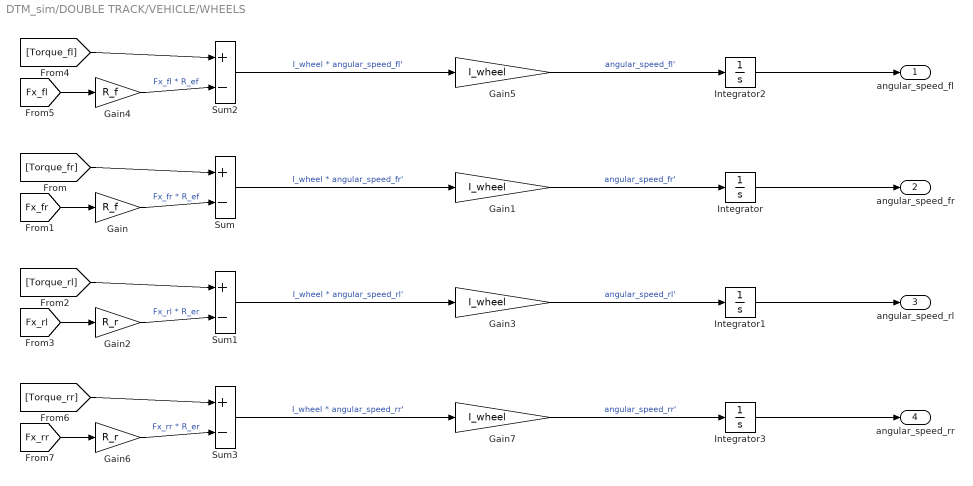
== system DTM_sim/DOUBLE TRACK/VEHICLE/WHEELS ==
  Gain : Gain  Gain=R_f
  Gain{1,3,5,7} (4 alike) : Gain  Gain=I_wheel
  Gain2 : Gain  Gain=R_r
  Gain4 : Gain  Gain=R_f
  Gain6 : Gain  Gain=R_r
  Integrator : Integrator  InitialCondition=angular_speed_fr0
  Integrator1 : Integrator  InitialCondition=angular_speed_rl0
  Integrator2 : Integrator  InitialCondition=angular_speed_fl0
  Integrator3 : Integrator  InitialCondition=angular_speed_rr0
  Sum{,1..3} (4 alike) : Sum  Inputs=|+|||-|
  angular_speed_fl : Outport
  angular_speed_fr : Outport  Port=2
  angular_speed_rl : Outport  Port=3
  angular_speed_rr : Outport  Port=4
  wires:
  [Torque_fr] -> Sum/1
  [Fx_fr] -> Gain/1
  Gain/1 -> Sum/2  "Fx_fr * R_ef"
  Sum/1 -> Gain1/1  "I_wheel * angular_speed_fr'"
  Gain1/1 -> Integrator/1  "angular_speed_fr'"
  Integrator/1 -> angular_speed_fr/1
  Gain2/1 -> Sum1/2  "Fx_rl * R_er"
  [Torque_rl] -> Sum1/1
  [Fx_rl] -> Gain2/1
  Sum1/1 -> Gain3/1  "I_wheel * angular_speed_rl'"
  Integrator1/1 -> angular_speed_rl/1
  Gain3/1 -> Integrator1/1  "angular_speed_rl'"
  Gain4/1 -> Sum2/2  "Fx_fl * R_ef"
  Gain5/1 -> Integrator2/1  "angular_speed_fl'"
  Sum2/1 -> Gain5/1  "I_wheel * angular_speed_fl'"
  Integrator2/1 -> angular_speed_fl/1
  [Torque_fl] -> Sum2/1
  [Fx_fl] -> Gain4/1
  Gain6/1 -> Sum3/2  "Fx_rr * R_er"
  [Torque_rr] -> Sum3/1
  Integrator3/1 -> angular_speed_rr/1
  Gain7/1 -> Integrator3/1  "angular_speed_rr'"
  [Fx_rr] -> Gain6/1
  Sum3/1 -> Gain7/1  "I_wheel * angular_speed_rr'"

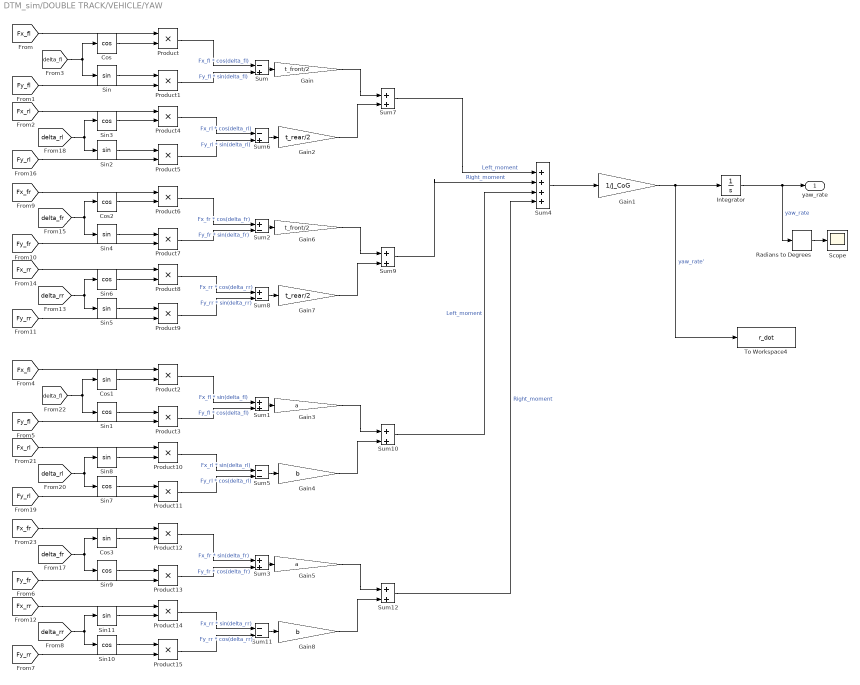
== system DTM_sim/DOUBLE TRACK/VEHICLE/YAW ==
  Cos : Trigonometry  Operator=cos
  Cos1 : Trigonometry
  Cos2 : Trigonometry  Operator=cos
  Cos3 : Trigonometry
  Gain : Gain  Gain=t_front/2
  Gain1 : Gain  Gain=1/J_CoG
  Gain2 : Gain  Gain=t_rear/2
  Gain3 : Gain  Gain=a
  Gain4 : Gain  Gain=b
  Gain5 : Gain  Gain=a
  Gain6 : Gain  Gain=t_front/2
  Gain7 : Gain  Gain=t_rear/2
  Gain8 : Gain  Gain=b
  Integrator : Integrator  InitialCondition=yaw_rate0
  Product{,1..15} (16 alike) : Product
  Radians to Degrees : simulink_extras/Transformations/Radians to Degrees
  Scope : Scope
  Sin{,2,4..5,8,11} (6 alike) : Trigonometry
  Sin{1,3,6..7,9..10} (6 alike) : Trigonometry  Operator=cos
  Sum : Sum  Inputs=-||+
  Sum1 : Sum  Inputs=+||+
  Sum{7,9..10,12} (4 alike) : Sum  Inputs=|+|||+|
  Sum11 : Sum  Inputs=-||-
  Sum2 : Sum  Inputs=+||-
  Sum3 : Sum  Inputs=+||+
  Sum4 : Sum  Inputs=|+|||+|||+|||+|
  Sum5 : Sum  Inputs=-||-
  Sum6 : Sum  Inputs=-||+
  Sum8 : Sum  Inputs=+||-
  To Workspace4 : ToWorkspace  VariableName=r_dot  SampleTime=-1
  yaw_rate : Outport
  wires:
  [Fx_fl] -> Product/1
  [Fy_rl] -> Product5/2
  [Fx_rl] -> Product4/1
  [delta_rl] -> Sin2/1, Sin3/1
  Cos/1 -> Product/2
  Sin2/1 -> Product5/1
  Sin3/1 -> Product4/2
  [Fy_fl] -> Product1/2
  Sin/1 -> Product1/1
  [delta_fl] -> Sin/1, Cos/1
  Product/1 -> Sum/1  "Fx_fl * cos(delta_fl)"
  Product1/1 -> Sum/2  "Fy_fl * sin(delta_fl)"
  Sum/1 -> Gain/1
  Sum6/1 -> Gain2/1
  Product4/1 -> Sum6/1  "Fx_rl * cos(delta_rl)"
  Product5/1 -> Sum6/2  "Fy_rl * sin(delta_rl)"
  Gain/1 -> Sum7/1
  Gain2/1 -> Sum7/2
  Sum7/1 -> Sum4/1  "Left_moment"
  Sum2/1 -> Gain6/1
  Product9/1 -> Sum8/2  "Fy_rr * sin(delta_rr)"
  Sum9/1 -> Sum4/2  "Right_moment"
  Product8/1 -> Sum8/1  "Fx_rr * cos(delta_rr)"
  Gain6/1 -> Sum9/1
  [delta_fr] -> Sin4/1, Cos2/1
  Sum8/1 -> Gain7/1
  Sin6/1 -> Product8/2
  Sin5/1 -> Product9/1
  Cos2/1 -> Product6/2
  [delta_rr] -> Sin5/1, Sin6/1
  [Fy_rr] -> Product9/2
  Product6/1 -> Sum2/1  "Fx_fr * cos(delta_fr)"
  [Fx_fr] -> Product6/1
  Product7/1 -> Sum2/2  "Fy_fr * sin(delta_fr)"
  Gain7/1 -> Sum9/2
  [Fx_rr] -> Product8/1
  [Fy_fr] -> Product7/2
  Sin4/1 -> Product7/1
  Sum4/1 -> Gain1/1
  Gain1/1 -> To Workspace4/1, Integrator/1  "yaw_rate'"
  Integrator/1 -> Radians to Degrees/1, yaw_rate/1  "yaw_rate"
  Cos3/1 -> Product12/2
  [delta_fr] -> Sin9/1, Cos3/1
  Product13/1 -> Sum3/2  "Fy_fr * cos(delta_fr)"
  Sum1/1 -> Gain3/1
  Sum3/1 -> Gain5/1
  Sin9/1 -> Product13/1
  Sum11/1 -> Gain8/1
  Sin8/1 -> Product10/2
  [Fy_rr] -> Product15/2
  Product15/1 -> Sum11/2  "Fy_rr * cos(delta_rr)"
  Sum10/1 -> Sum4/3  "Left_moment"
  [Fy_fr] -> Product13/2
  Gain5/1 -> Sum12/1
  Product14/1 -> Sum11/1  "Fx_rr * sin(delta_rr)"
  [Fx_rr] -> Product14/1
  Sin11/1 -> Product14/2
  Gain8/1 -> Sum12/2
  [Fx_fr] -> Product12/1
  Cos1/1 -> Product2/2
  [Fy_rl] -> Product11/2
  Gain4/1 -> Sum10/2
  Product12/1 -> Sum3/1  "Fx_fr * sin(delta_fr)"
  [delta_rr] -> Sin10/1, Sin11/1
  [Fx_rl] -> Product10/1
  [Fx_fl] -> Product2/1
  Gain3/1 -> Sum10/1
  Sum12/1 -> Sum4/4  "Right_moment"
  Sum5/1 -> Gain4/1
  Sin10/1 -> Product15/1
  Sin1/1 -> Product3/1
  Product2/1 -> Sum1/1  "Fx_fl * sin(delta_fl)"
  Product11/1 -> Sum5/2  "Fy_rl * cos(delta_rl)"
  [Fy_fl] -> Product3/2
  Product3/1 -> Sum1/2  "Fy_fl * cos(delta_fl)"
  Product10/1 -> Sum5/1  "Fx_rl * sin(delta_rl)"
  [delta_fl] -> Sin1/1, Cos1/1
  Sin7/1 -> Product11/1
  [delta_rl] -> Sin7/1, Sin8/1
  Radians to Degrees/1 -> Scope/1

== matlab function DTM_sim/DOUBLE TRACK/TIRES/TIRES ==
  data: alpha_fl input; alpha_fr input; alpha_rl input; alpha_rr input; Fz_fl input; Fz_fr input; Fz_rl input; Fz_rr input; Fxfl input; Fxfr input; Fxrl input; Fxrr input; F_xfl output; F_xfr output; F_xrl output; F_xrr output; F_yfl output; F_yfr output; F_yrl output; F_yrr output
function [F_xfl,F_xfr,F_xrl,F_xrr,F_yfl,F_yfr,F_yrl,F_yrr] = fcn(alpha_fl,alpha_fr,alpha_rl,alpha_rr,Fz_fl,Fz_fr,Fz_rl,Fz_rr,Fxfl,Fxfr,Fxrl,Fxrr) 
%% Separation of inputs variable
% alpha_fl = inputs(1); % [rad]
% alpha_fr = inputs(2); % [rad]
% 
% alpha_rl  = inputs(3); % [rad]
% alpha_rr  = inputs(4); % [rad]
% 
% Fxfl = inputs(5); % [N] longitudinal left frontal force
% Fxfr = inputs(6); % [N] longitudinal right frontal force
% 
% Fxrl  = inputs(7); % [N] longitudinal left rear force
% Fxrr  = inputs(8); % [N] longitudinal right rear force
% 
% Fz_fl = inputs(9); % [N] vertical load on front axle
% Fz_fr = inputs(10); % [N] vertical load on front axle
% 
% Fz_rl = inputs(11); % [N] vertical load on rear axle
% Fz_rr = inputs(12); % [N] vertical load on rear axle
% 
% Fxrl_LQR = inputs(13); % [N] correction on longitudinal left rear force given by LQR
% Fxrr_LQR = inputs(14); % [N] correction on longitudinal right rear force given by LQR

%% Maximum saturation and Stiffness
F_ymax = @(mu,Fz,Fx) sqrt((mu*Fz)^2-Fx^2);

alpha_s= @(Fy_max,C_alpha) atan((3*Fy_max)/C_alpha); % [rad] maximum slip angle beyond which tire starts to slide

Cy_front  = 370.36; %[N/rad] Cornering stiffness front tyre
Cy_rear   = 1134.05;%[N/rad] Cornering stiffness rear tyre

mu_front  = 0.5;
mu_rear   = 0.47;

%% Longitudinal forces 

F_xfl = Fxfl; % [N] 
F_xfr = Fxfr; % [N] 

F_xrl = Fxrl; % [N] 
F_xrr = Fxrr; % [N] 

% saturation of the tire
if abs(F_xrl) > mu_rear*Fz_rl - 0.0001
    F_xrl = (mu_rear*Fz_rl - 0.0001)*sign(F_xrl);
end

if abs(F_xrr) > mu_rear*Fz_rr - 0.0001
    F_xrr = (mu_rear*Fz_rr - 0.0001)*sign(F_xrr);
end

F_ymaxrear_l = F_ymax(mu_rear,Fz_rl,F_xrl);
F_ymaxrear_r = F_ymax(mu_rear,Fz_rr,F_xrr);

F_ymaxfront_l= F_ymax(mu_front,Fz_fl,F_xfl);
F_ymaxfront_r= F_ymax(mu_front,Fz_fr,F_xfr);

%% Lateral forces 
Fy_fiala = @(Fy_max,Cy,mu,alpha) Cy*tan(alpha)- ...
                                        Cy^2./(3*Fy_max).*abs(tan(alpha)).*tan(alpha)+ ...
                                        Cy^3./(27*(Fy_max)^2).*(tan(alpha)).^3; 


%________ FRONT
if abs(alpha_fl)>=alpha_s(F_ymaxfront_l,Cy_front/2)
    F_yfl = F_ymaxfront_l*sign(alpha_fl);
else
    F_yfl = Fy_fiala(F_ymaxfront_l,Cy_front/2,mu_front,abs(alpha_fl))*sign(alpha_fl);
end

if abs(alpha_fr)>=alpha_s(F_ymaxfront_r,Cy_front/2)
    F_yfr = F_ymaxfront_r*sign(alpha_fr);
else
    F_yfr = Fy_fiala(F_ymaxfront_r,Cy_front/2,mu_front,abs(alpha_fr))*sign(alpha_fr);
end
%________ REAR
if abs(alpha_rl)>=alpha_s(F_ymaxrear_l,Cy_rear/2)
    F_yrl = F_ymaxrear_l*sign(alpha_rl);
else
    F_yrl = Fy_fiala(F_ymaxrear_l,Cy_rear/2,mu_rear,abs(alpha_rl))*sign(alpha_rl);
end

if abs(alpha_rr)>=alpha_s(F_ymaxrear_r,Cy_rear/2)
    F_yrr = F_ymaxrear_r*sign(alpha_rr);
else
    F_yrr = Fy_fiala(F_ymaxrear_r,Cy_rear/2,mu_rear,abs(alpha_rr))*sign(alpha_rr);
end
